simulink model "model_3"  (R2018b)
settings: Solver=VariableStepAuto  StartTime=0.0  StopTime=1  RelTol=1e-6
StopFcn:
  | location = 150;
  | fault = 999910;
  | voltage = Vm(:,2:4);
  | voltage(:,4:6) = Vp(:,2:4);
  | current = Im(:,2:4);
  | current(:,4:6) = Ip(:,2:4);
  | current(:,7) = fault;
  | current(:,8) = location;
  | logg = [voltage,current];
  | data = xlsread('fdata3');
  | data = [data;logg];
  | xlswrite('fdata3',data);
undefined symbols (not defined in the file): Angle, Magnitude
libraries: powerlib x7, powerlib_meascontrol x2
settings Model: Creator=Edagotti Pavankumar  LastModifiedBy=dedeepya
settings SolverCC: ZeroCrossAlgorithm=Adaptive
settings DebuggingCC: IgnoredZcDiagnostic=none

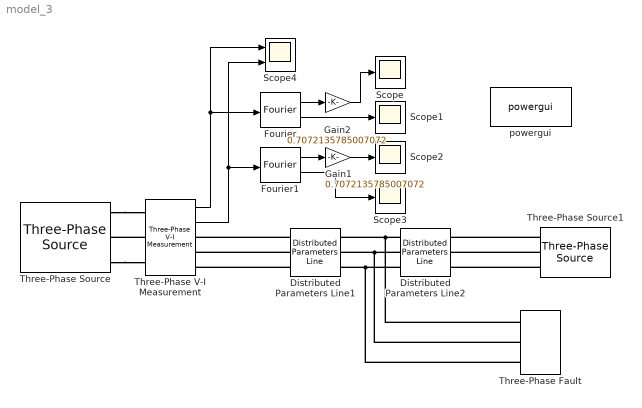
== system model_3 ==
  Distributed Parameters Line1 : powerlib/Elements/Distributed Parameters Line  Phases=3  Frequency=50  Resistance=[0.0238 0.3885]  Inductance="[9.5095e-4  3.25089e-3]"  Capacitance=[12.74e-9 7.751e-9]  Length=150  x1=[1.37715638489664e-10 215991.177629105 215991.177629105;314.159265358979 314.159265358979 314.159265358979;3.1179819917031 1.00925112695349 -0.561545199841409]  x2=[8.48515176744739e-11 211001.309712381 211001.309712381;314.159265358979 314.159265358979 314.159265358979;1.87466681559939 0.555361583254945 -1.01543474353995]  x3=[7.06448823707835e-13 1358.35479564109 1358.35479564109;314.159265358979 314.159265358979 314.159265358979;-0.236549011466092 -2.39788057268035 2.31450840770434]  x4=[4.3473773766636e-13 2870.80842105717 2870.80842105717;314.159265358979 314.159265358979 314.159265358979;2.9050436421237 0.722114240717427 -0.84868208607747]  x5=0.0007529588891666  V1=[1.377e-10 2.16e+05 2.16e+05;314.2 314.2 314.2;3.118 1.009 -0.5615]  V2=[8.485e-11 2.11e+05 2.11e+05;314.2 314.2 314.2;1.875 0.5554 -1.015]  I1=[7.064e-13 1358 1358;314.2 314.2 314.2;-0.2365 -2.398 2.315]  I2=[4.347e-13 2871 2871;314.2 314.2 314.2;2.905 0.7221 -0.8487]  nHarmo=1  Measurements=None
      settings: SourceProductName=Simscape Power Systems
  Distributed Parameters Line2 : powerlib/Elements/Distributed Parameters Line  Phases=3  Frequency=50  Resistance=[0.0238 0.3885]  Inductance="[9.5095e-4  3.25089e-3]"  Capacitance=[12.74e-9 7.751e-9]  Length=50  x1=[8.67793310453749e-11 211001.309712381 211001.309712381;314.159265358979 314.159265358979 314.159265358979;2.06832187689738 0.664710233858622 -0.906086092936275]  x2=[9.11674875980073e-11 217679.745974723 217679.745974723;314.159265358979 314.159265358979 314.159265358979;2.56339626142097 0.519061865430636 -1.05173446136426]  x3=[2.50427424250028e-12 1390.19758440377 1390.19758440376;314.159265358979 314.159265358979 314.159265358979;-1.46979249749112 -2.12543956014665 2.58694942023805]  x4=[1.11994548810648e-12 2875.54915886328 2875.54915886327;314.159265358979 314.159265358979 314.159265358979;-2.29314710607688 0.776483171848123 -0.794313154946772]  x5=0.000250986296388867  V1=[8.678e-11 2.11e+05 2.11e+05;314.2 314.2 314.2;2.068 0.6647 -0.9061]  V2=[9.117e-11 2.177e+05 2.177e+05;314.2 314.2 314.2;2.563 0.5191 -1.052]  I1=[2.504e-12 1390 1390;314.2 314.2 314.2;-1.47 -2.125 2.587]  I2=[1.12e-12 2876 2876;314.2 314.2 314.2;-2.293 0.7765 -0.7943]  nHarmo=1  Measurements=None
      settings: SourceProductName=Simscape Power Systems
  Fourier : powerlib_meascontrol/Measurements/Fourier  Freq=50  n=1  InInit=[0, 0]  Ts=0
      settings: SourceProductName=Simscape Power Systems
  Fourier1 : powerlib_meascontrol/Measurements/Fourier  Freq=50  n=1  InInit=[0, 0]  Ts=0
      settings: SourceProductName=Simscape Power Systems
  Gain1 : Gain  Gain=0.7072135785007072
  Gain2 : Gain  Gain=0.7072135785007072
  Scope{,1..3} (4 alike) : Scope
  Scope4 : Scope  NumInputPorts=2
  Three-Phase V-I Measurement : powerlib/Measurements/Three-Phase V-I Measurement  VoltageMeasurement=phase-to-ground  SetLabelV=off  LabelV=Vabc  Vpu=on  VpuLL=off  CurrentMeasurement=yes  SetLabelI=off  LabelI=Iabc  Ipu=on  Pbase=100e6  Vbase=220e3  OutputType=Magnitude-Angle  PhasorSimulation=off  PSBequivalent=0
  Three-Phase Fault : powerlib/Elements/Three-Phase Fault  InitialStates=0  FaultA=on  FaultB=on  FaultC=on  GroundFault=off  SwitchTimes=0.5  External=off  SwitchStatus=NaN  FaultResistance=20  GroundResistance=0.001  SnubberResistance=1e6  SnubberCapacitance=inf  Measurements=None
  Three-Phase Source : powerlib/Electrical Sources/Three-Phase Source  InternalConnection=Yg  VoltagePhases=off  Voltage=220e3  PhaseAngle=40  Voltage_phases=[25e3 25e3 25e3]/sqrt(3)  PhaseAngles_phases=[0 -120 +120]  Frequency=50  NonIdealSource=on  SpecifyImpedance=off  Resistance=0.8929  Inductance=16.58e-3  ShortCircuitLevel=170e6  BaseVoltage=220e3  XRratio=7  BusType=swing  Pref=10e3  Qref=0  Prefabc=[10e3, 10e3, 10e3]  Qrefabc=[0, 0, 0]  Qmin=-inf  Qmax=inf
  Three-Phase Source1 : powerlib/Electrical Sources/Three-Phase Source  InternalConnection=Yg  VoltagePhases=off  Voltage=220e3  PhaseAngle=0  Voltage_phases=[25e3 25e3 25e3]/sqrt(3)  PhaseAngles_phases=[0 -120 +120]  Frequency=50  NonIdealSource=on  SpecifyImpedance=off  Resistance=0.8929  Inductance=16.58e-3  ShortCircuitLevel=176e6  BaseVoltage=220e3  XRratio=7  BusType=swing  Pref=inf  Qref=inf  Prefabc=[10e3, 10e3, 10e3]  Qrefabc=[0, 0, 0]  Qmin=-inf  Qmax=inf
  powergui : powerlib/powergui  Priority=1  SimulationMode=Continuous  SampleTime=50e-10  frequency=50  Iterations=50  frequencyindice=50  Pbase=100e6  ErrMax=1e-4  UnitsV=kV  UnitsW=MW  buscounter=0  FunctionMessages=off  echomessages=off  EnableUseOfTLC=off  CurrentSourceSwitches=off  DisableSnubberDevices=off  DisableRonSwitches=off  DisableVfSwitches=off  DisplayEquations=off  SolverType=Tustin/Backward Euler (TBE)  Interpol=off  ExternalGateDelay=off  methode=off  Ts=100  x0status=blocks  SPID=off  SwTol=0  HookPort=off  RestoreLinks=warning  ResistiveCurrentMeasurement=off  Frange=[0:2:500]  Ylog=off  Xlog=on  ShowGrid=off  save=off  variable=ZData  structure=0  ZoomFFT=off  StartTime=0.0  cycles=1  DisplayStyle=1  fundamental=60  FreqAxis=off  MaxFrequency=1000  frequencyindicesteady=1  RmsSteady=2  display=off
  wires:
  Three-Phase V-I Measurement/1 -> Scope4/1, Fourier/1
  Fourier1/2 -> Scope3/1
  Three-Phase V-I Measurement/2 -> Scope4/2, Fourier1/1
  Fourier/2 -> Scope1/1
  Gain1/1 -> Scope2/1
  Fourier1/1 -> Gain1/1
  Gain2/1 -> Scope/1
  Fourier/1 -> Gain2/1
  connections:
  Three-Phase V-I Measurement/LConn2 -- Three-Phase Source/RConn2
  Three-Phase Source/RConn1 -- Three-Phase V-I Measurement/LConn1
  Three-Phase Source/RConn3 -- Three-Phase V-I Measurement/LConn3
  Distributed Parameters Line1/LConn1 -- Three-Phase V-I Measurement/RConn1
  Distributed Parameters Line1/LConn2 -- Three-Phase V-I Measurement/RConn2
  Distributed Parameters Line1/LConn3 -- Three-Phase V-I Measurement/RConn3
  Distributed Parameters Line2/LConn1 -- Three-Phase Fault/LConn1 -- Distributed Parameters Line1/RConn1
  Distributed Parameters Line2/LConn2 -- Three-Phase Fault/LConn2 -- Distributed Parameters Line1/RConn2
  Distributed Parameters Line2/LConn3 -- Three-Phase Fault/LConn3 -- Distributed Parameters Line1/RConn3
  Three-Phase Source1/RConn1 -- Distributed Parameters Line2/RConn1
  Three-Phase Source1/RConn2 -- Distributed Parameters Line2/RConn2
  Three-Phase Source1/RConn3 -- Distributed Parameters Line2/RConn3
